simulink subsystem "PvtSubSys_VSM_LKA"  (R2020b)
settings: Solver=VariableStepAuto  StartTime=0.0  StopTime=10.0  RelTol=1e-3
values from neighbouring files (symbols this model uses):
  P_VSM_LKA_AbsEspInTime = 3.0    [LKA.sldd]
  P_VSM_LKA_absLongitudeAcceIn = 2.5    [LKA.sldd]
  P_VSM_LKA_absLongitudeAcceInTime = 3.0    [LKA.sldd]
  P_VSM_LKA_absLongitudeAcceOut = 3.0    [LKA.sldd]
  P_VSM_LKA_AccPedalPosnOut = 30.0    [LKA.sldd]
  P_VSM_LKA_AccPedalRateOutTime = 0.0    [LKA.sldd]
  P_VSM_LKA_AccRateIn = 30.0    [LKA.sldd]
  P_VSM_LKA_AccRateInTime = 1.5    [LKA.sldd]
  P_VSM_LKA_AccRateOut = 70.0    [LKA.sldd]
  P_VSM_LKA_BrakePressIn = 3.0    [LKA.sldd]
  P_VSM_LKA_BrakePressInTime = 1.5    [LKA.sldd]
  P_VSM_LKA_BrakePressOut = 5.0    [LKA.sldd]
  P_VSM_LKA_CurveFactor = 1.0    [LKA.sldd]
  P_VSM_LKA_DriverInputTrqValueIn = 2.0    [LKA.sldd]
  P_VSM_LKA_DriverInputTrqValueInTime = 3.0    [LKA.sldd]
  P_VSM_LKA_DriverInputTrqValueOut = 2.3    [LKA.sldd]
  P_VSM_LKA_EndSwitch = 1.0    [LKA.sldd]
  P_VSM_LKA_LaneChangeOffset = 0.11    [LKA.sldd]
  P_VSM_LKA_LaneCurveIn = 0.005    [LKA.sldd]
  P_VSM_LKA_LaneCurveOut = 0.006    [LKA.sldd]
  P_VSM_LKA_LateralAcceIn = 3.0    [LKA.sldd]
  P_VSM_LKA_LateralAcceInTime = 3.0    [LKA.sldd]
  P_VSM_LKA_LateralAcceOut = 3.5    [LKA.sldd]
  P_VSM_LKA_LongitudeAcceIn = 3.0    [LKA.sldd]
  P_VSM_LKA_LongitudeAcceOut = 3.5    [LKA.sldd]
  P_VSM_LKA_OverrideInTime = 1.5    [LKA.sldd]
  P_VSM_LKA_OverrideTime = 0.3    [LKA.sldd]
  P_VSM_LKA_OverrideValue = 1.2    [LKA.sldd]
  P_VSM_LKA_State_Absesp_enable = 1.0    [LKA.sldd]
  P_VSM_LKA_State_Accpedalrate_enable = 1.0    [LKA.sldd]
  P_VSM_LKA_State_Breakpressure_enable = 1.0    [LKA.sldd]
  P_VSM_LKA_State_DriverInputTrqValue_enable = 1.0    [LKA.sldd]
  P_VSM_LKA_State_Eps_enable = 1.0    [LKA.sldd]
  P_VSM_LKA_State_ESSSts_enable = 1.0    [LKA.sldd]
  P_VSM_LKA_State_Failsafe_enable = 1.0    [LKA.sldd]
  P_VSM_LKA_State_GEAR_enable = 1.0    [LKA.sldd]
  P_VSM_LKA_State_Handson_enable = 1.0    [LKA.sldd]
  P_VSM_LKA_State_Headingangle_enable = 1.0    [LKA.sldd]
  P_VSM_LKA_State_Lane_enable = 1.0    [LKA.sldd]
  P_VSM_LKA_State_LaneChange_enable = 1.0    [LKA.sldd]
  P_VSM_LKA_State_Lanecurve_enable = 1.0    [LKA.sldd]
  P_VSM_LKA_State_LateralAcce_enable = 1.0    [LKA.sldd]
  P_VSM_LKA_State_LongitudeAcc_enable = 1.0    [LKA.sldd]
  P_VSM_LKA_State_Overide_enable = 1.0    [LKA.sldd]
  P_VSM_LKA_State_Param_AngleOffset = 0.15    [LKA.sldd]
  P_VSM_LKA_State_Param_InterventionZoneIn = 0.4    [LKA.sldd]
  P_VSM_LKA_State_Param_InterventionZoneOut = -0.65    [LKA.sldd]
  P_VSM_LKA_State_Param_LaneCurve : value not decoded    [LKA.sldd]
  P_VSM_LKA_State_Param_LaneCurve_Offset : value not decoded    [LKA.sldd]
  P_VSM_LKA_State_Param_LaneWidth_Offset : value not decoded    [LKA.sldd]
  P_VSM_LKA_State_Param_OutOffset = 0.2    [LKA.sldd]
  P_VSM_LKA_State_Param_REInterventionZoneIn = 0.55    [LKA.sldd]
  P_VSM_LKA_State_Param_Sensitive_Offset : value not decoded    [LKA.sldd]
  P_VSM_LKA_State_SteerWheelAngle_enable = 1.0    [LKA.sldd]
  P_VSM_LKA_State_SteerWheelSpd_enable = 1.0    [LKA.sldd]
  P_VSM_LKA_State_TJASts_enable = 1.0    [LKA.sldd]
  P_VSM_LKA_State_TurnLight_enable = 1.0    [LKA.sldd]
  P_VSM_LKA_State_Vehspeed_enable = 1.0    [LKA.sldd]
  P_VSM_LKA_State_Yawsup_enable = 1.0    [LKA.sldd]
  P_VSM_LKA_SteerWheelAngleIn = 70.0    [LKA.sldd]
  P_VSM_LKA_SteerWheelAngleInTime = 3.0    [LKA.sldd]
  P_VSM_LKA_SteerWheelAngleOut = 90.0    [LKA.sldd]
  P_VSM_LKA_SteerWheelSpdIn = 150.0    [LKA.sldd]
  P_VSM_LKA_SteerWheelSpdInTime = 3.0    [LKA.sldd]
  P_VSM_LKA_SteerWheelSpdOut = 200.0    [LKA.sldd]
  P_VSM_LKA_TurnLightInTime = 3.0    [LKA.sldd]
  P_VSM_LKA_Warnarea1 = -0.55    [LKA.sldd]
  P_VSM_LKA_Warnarea2 = -0.35    [LKA.sldd]
  P_VSM_LKA_WarnInTime = 2.0    [LKA.sldd]
  P_VSM_LKA_WhelDy = 2.0    [LKA.sldd]
  P_VSM_LKA_YawRateIn = 0.2    [LKA.sldd]
  P_VSM_LKA_YawRateInTime = 1.0    [LKA.sldd]
  P_VSM_LKA_YawRateOut = 0.25    [LKA.sldd]
undefined symbols (not defined in the file or in its folder): P_VSM_LKA_AddOffset, P_VSM_LSMC_SampleTime, STATE
libraries: simulink x162
(part 4 of 5)

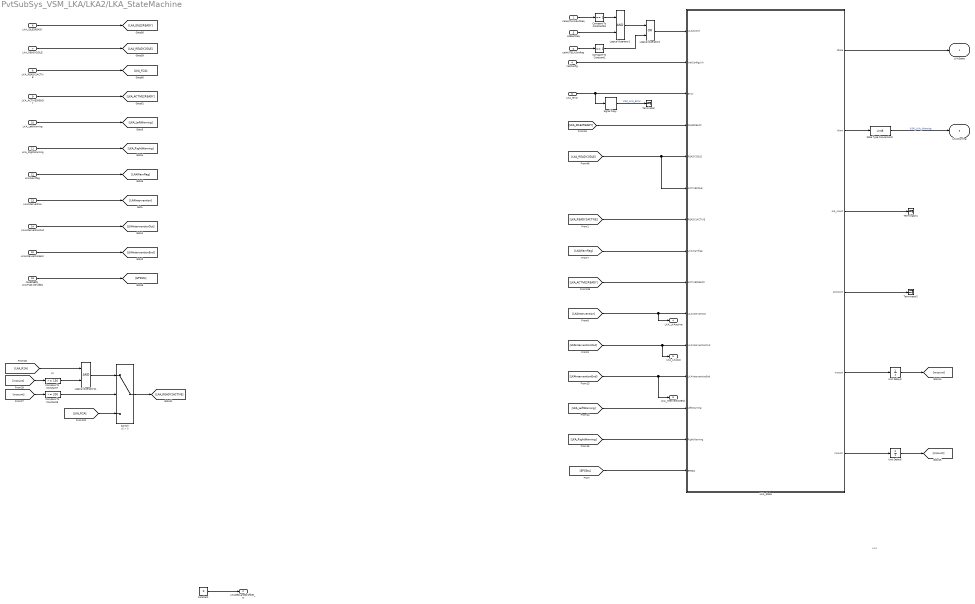
== system PvtSubSys_VSM_LKA/LKA2/LKA_StateMachine ==
  note: 3S
  note: LKA
  canHUTLKASwtReq : Inport
  canHUTELKSwtReq : Inport  Port=2
  LSSSwtReq : Inport  Port=3
  VehConfig : Inport  Port=4
  LKA_Error : Inport  Port=5
  LKA_IDLE2READY : Inport  Port=6
  LKA_READY2IDLE : Inport  Port=7
  LKA_READY2ACTIVE : Inport  Port=8
  LKA_ACTIVE2READY : Inport  Port=9
  LKA_LeftWarning : Inport  Port=10
  LKA_RightWarning : Inport  Port=11
  LKAWarnflag : Inport  Port=12
  LKAIntervention : Inport  Port=13
  LKAInterventionOut : Inport  Port=14
  LKAInterventionEnd : Inport  Port=15
  canEPSEPS_LKATrqOvlDlvdSts : Inport  Port=16
  Compare To Constant1 : simulink/Logic and Bit Operations/Compare To Constant  relop===  const=1  OutDataTypeStr=boolean
  Compare To Constant53 : simulink/Logic and Bit Operations/Compare To Constant  relop===  const=1  OutDataTypeStr=boolean
  Compare To Constant6 : simulink/Logic and Bit Operations/Compare To Constant  relop=>=  const=200  OutDataTypeStr=boolean
  Compare To Constant7 : simulink/Logic and Bit Operations/Compare To Constant  relop=>=  const=150  OutDataTypeStr=boolean
  Constant : Constant  Value=0
  Data Type Conversion2 : DataTypeConversion  OutDataTypeStr=uint8
  LKA_State : Stateflow chart  TreatAsAtomicUnit=on
  Logical Operator1 : Logic  AllPortsSameDT=off  OutDataTypeStr=boolean
  Logical Operator11 : Logic  AllPortsSameDT=off  OutDataTypeStr=boolean
  Logical Operator2 : Logic  Operator=OR  AllPortsSameDT=off  OutDataTypeStr=boolean
  Signal Copy : SignalConversion  OverrideOpt=off
  Switch : Switch  Criteria=u2 > Threshold
  Terminator : Terminator
  Terminator1 : Terminator
  Terminator2 : Terminator
  Unit Delay3 : UnitDelay  SampleTime=-1  HasFrameUpgradeWarning=on
  Unit Delay6 : UnitDelay  SampleTime=-1  HasFrameUpgradeWarning=on
  LKAState : Outport
  LKADesLaneDyoffset_m : Outport  Port=2
  LKAWarning : Outport  Port=3
  LKA_LKAactive : Outport  Port=4
  LKA_LKAout : Outport  Port=5
  LKA_InterventionEnd : Outport  Port=6
  wires:
  Signal Copy/1 -> Terminator/1  "VSM_LKA_Error"
  [EPSSts] -> LKA_State/15(EPSSts)
  canEPSEPS_LKATrqOvlDlvdSts/1 -> [EPSSts]
  LSSSwtReq/1 -> Logical Operator1/2
  Logical Operator2/1 -> LKA_State/1(LKASwitch)
  LKAInterventionEnd/1 -> [LKAInterventionEnd]
  LKAInterventionOut/1 -> [LKAInterventionOut]
  LKAIntervention/1 -> [LKAIntervention]
  LKAWarnflag/1 -> [LKAWarnflag]
  LKA_RightWarning/1 -> [LKA_RightWarning]
  LKA_LeftWarning/1 -> [LKA_LeftWarning]
  Switch/1 -> [LKA_READY2ACTIVE]
  [LKAInterventionEnd] -> LKA_State/12(LKAInterventionEnd), LKA_InterventionEnd/1
  [LKAInterventionOut] -> LKA_State/11(LKAInterventionOut), LKA_LKAout/1
  [LKAIntervention] -> LKA_LKAactive/1, LKA_State/10(LKAIntervention)
  [LKAWarnflag] -> LKA_State/8(LKAWarnflag)
  LKA_State/1(State) -> LKAState/1
  Data Type Conversion2/1 -> LKAWarning/1  "VSM_LKA_Warning"
  LKA_State/4(actcount) -> Terminator2/1
  LKA_State/3(out_count) -> Terminator1/1
  Compare To Constant1/1 -> Logical Operator2/2
  Constant/1 -> LKADesLaneDyoffset_m/1
  [LKA_ACTIVE2READY] -> LKA_State/9(ACTIVE2READY)
  LKA_Error/1 -> LKA_State/3(Error), Signal Copy/1
  [LKA_RightWarning] -> LKA_State/14(RightWarning)
  canHUTLKASwtReq/1 -> Compare To Constant53/1
  [LKA_LeftWarning] -> LKA_State/13(LeftWarning)
  LKA_State/2(Warn) -> Data Type Conversion2/1
  LKA_IDLE2READY/1 -> [LKA_IDLE2READY]
  LKA_READY2IDLE/1 -> [LKA_READY2IDLE]
  LKA_READY2ACTIVE/1 -> [LKA_R2A]
  LKA_ACTIVE2READY/1 -> [LKA_ACTIVE2READY]
  [LKA_IDLE2READY] -> LKA_State/4(IDLE2READY)
  Compare To Constant53/1 -> Logical Operator1/1
  [LKA_READY2IDLE] -> LKA_State/5(READY2IDLE), LKA_State/6(ACTIVE2IDLE)
  LKA_State/5(wcount) -> Unit Delay3/1
  [LKA_R2A] -> Switch/3
  [LKA_READY2ACTIVE] -> LKA_State/7(READY2ACTIVE)
  [LKA_R2A] -> Logical Operator11/1
  Logical Operator11/1 -> Switch/1
  [wcount] -> Compare To Constant6/1
  Compare To Constant6/1 -> Switch/2
  LKA_State/6(incount) -> Unit Delay6/1
  Compare To Constant7/1 -> Logical Operator11/2
  [incount] -> Compare To Constant7/1
  Unit Delay3/1 -> [wcount]
  Unit Delay6/1 -> [incount]
  canHUTELKSwtReq/1 -> Compare To Constant1/1
  Logical Operator1/1 -> Logical Operator2/1
  VehConfig/1 -> LKA_State/2(VehConfigLKA)

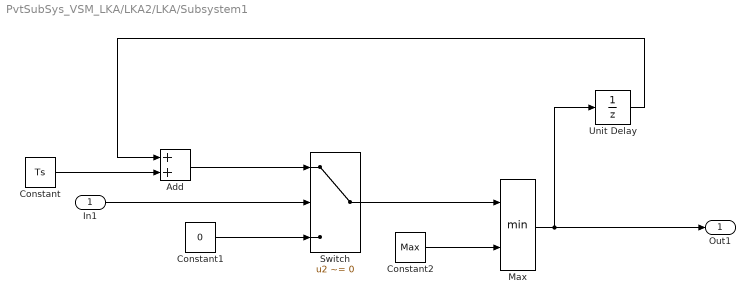
== system PvtSubSys_VSM_LKA/LKA2/LKA/Subsystem1 ==
  In1 : Inport
  Add : Sum
  Constant : Constant  Value=Ts
  Constant1 : Constant  Value=0
  Constant2 : Constant  Value=Max
  Max : MinMax  Inputs=2
  Switch : Switch  Criteria=u2 ~= 0
  Unit Delay : UnitDelay  SampleTime=-1  HasFrameUpgradeWarning=on
  Out1 : Outport
  wires:
  Unit Delay/1 -> Add/1
  In1/1 -> Switch/2
  Constant/1 -> Add/2
  Constant1/1 -> Switch/3
  Add/1 -> Switch/1
  Max/1 -> Unit Delay/1, Out1/1
  Constant2/1 -> Max/2
  Switch/1 -> Max/1

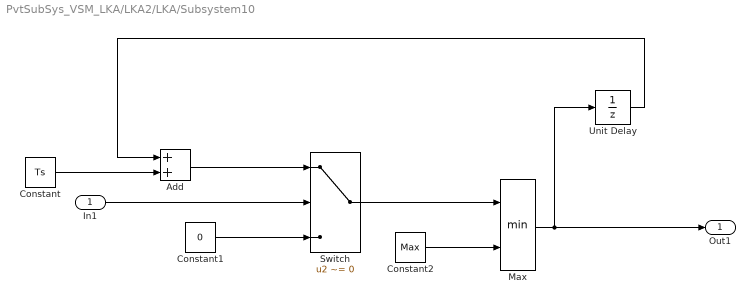
== system PvtSubSys_VSM_LKA/LKA2/LKA/Subsystem10 ==
  In1 : Inport
  Add : Sum
  Constant : Constant  Value=Ts
  Constant1 : Constant  Value=0
  Constant2 : Constant  Value=Max
  Max : MinMax  Inputs=2
  Switch : Switch  Criteria=u2 ~= 0
  Unit Delay : UnitDelay  SampleTime=-1  HasFrameUpgradeWarning=on
  Out1 : Outport
  wires:
  Switch/1 -> Max/1
  Constant2/1 -> Max/2
  Max/1 -> Out1/1, Unit Delay/1
  Add/1 -> Switch/1
  Constant1/1 -> Switch/3
  Constant/1 -> Add/2
  In1/1 -> Switch/2
  Unit Delay/1 -> Add/1

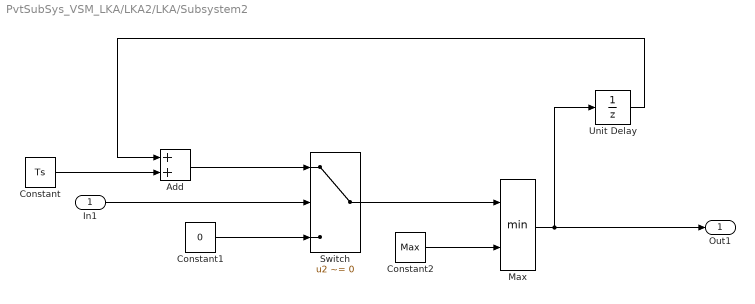
== system PvtSubSys_VSM_LKA/LKA2/LKA/Subsystem2 ==
  In1 : Inport
  Add : Sum
  Constant : Constant  Value=Ts
  Constant1 : Constant  Value=0
  Constant2 : Constant  Value=Max
  Max : MinMax  Inputs=2
  Switch : Switch  Criteria=u2 ~= 0
  Unit Delay : UnitDelay  SampleTime=-1  HasFrameUpgradeWarning=on
  Out1 : Outport
  wires:
  Unit Delay/1 -> Add/1
  In1/1 -> Switch/2
  Constant/1 -> Add/2
  Constant1/1 -> Switch/3
  Add/1 -> Switch/1
  Max/1 -> Unit Delay/1, Out1/1
  Constant2/1 -> Max/2
  Switch/1 -> Max/1

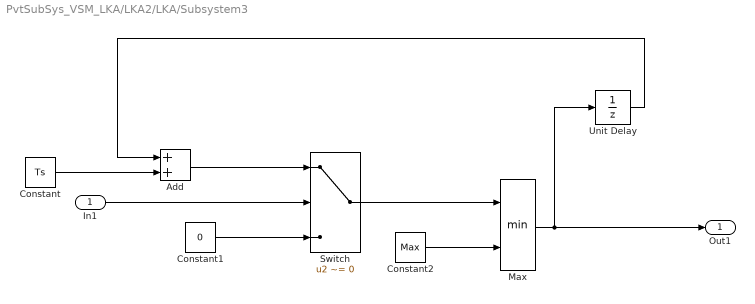
== system PvtSubSys_VSM_LKA/LKA2/LKA/Subsystem3 ==
  In1 : Inport
  Add : Sum
  Constant : Constant  Value=Ts
  Constant1 : Constant  Value=0
  Constant2 : Constant  Value=Max
  Max : MinMax  Inputs=2
  Switch : Switch  Criteria=u2 ~= 0
  Unit Delay : UnitDelay  SampleTime=-1  HasFrameUpgradeWarning=on
  Out1 : Outport
  wires:
  Switch/1 -> Max/1
  Constant2/1 -> Max/2
  Max/1 -> Out1/1, Unit Delay/1
  Add/1 -> Switch/1
  Constant1/1 -> Switch/3
  Constant/1 -> Add/2
  In1/1 -> Switch/2
  Unit Delay/1 -> Add/1

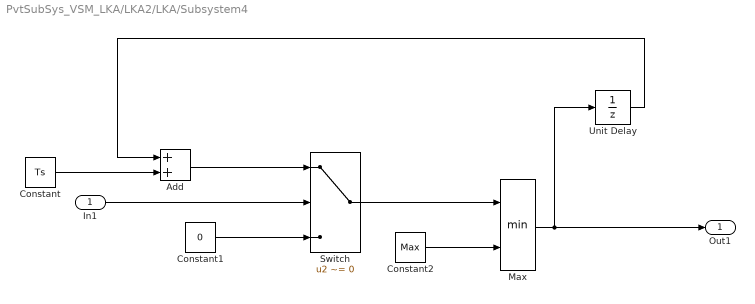
== system PvtSubSys_VSM_LKA/LKA2/LKA/Subsystem4 ==
  In1 : Inport
  Add : Sum
  Constant : Constant  Value=Ts
  Constant1 : Constant  Value=0
  Constant2 : Constant  Value=Max
  Max : MinMax  Inputs=2
  Switch : Switch  Criteria=u2 ~= 0
  Unit Delay : UnitDelay  SampleTime=-1  HasFrameUpgradeWarning=on
  Out1 : Outport
  wires:
  Switch/1 -> Max/1
  Constant2/1 -> Max/2
  Max/1 -> Out1/1, Unit Delay/1
  Add/1 -> Switch/1
  Constant1/1 -> Switch/3
  Constant/1 -> Add/2
  In1/1 -> Switch/2
  Unit Delay/1 -> Add/1

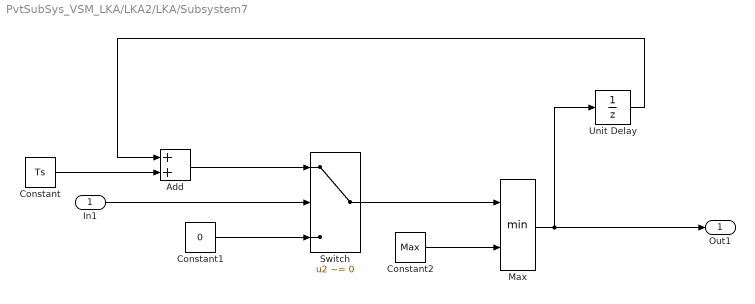
== system PvtSubSys_VSM_LKA/LKA2/LKA/Subsystem7 ==
  In1 : Inport
  Add : Sum
  Constant : Constant  Value=Ts
  Constant1 : Constant  Value=0
  Constant2 : Constant  Value=Max
  Max : MinMax  Inputs=2
  Switch : Switch  Criteria=u2 ~= 0
  Unit Delay : UnitDelay  SampleTime=-1  HasFrameUpgradeWarning=on
  Out1 : Outport
  wires:
  Unit Delay/1 -> Add/1
  In1/1 -> Switch/2
  Constant/1 -> Add/2
  Constant1/1 -> Switch/3
  Add/1 -> Switch/1
  Max/1 -> Unit Delay/1, Out1/1
  Constant2/1 -> Max/2
  Switch/1 -> Max/1

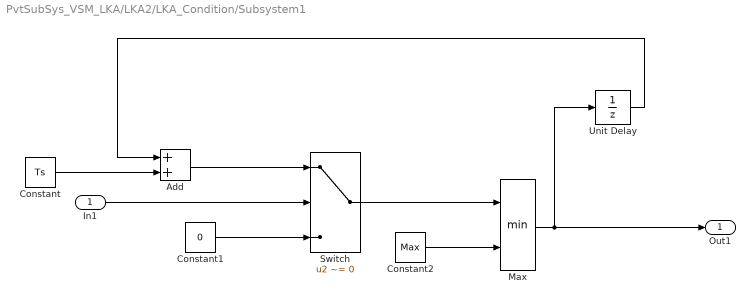
== system PvtSubSys_VSM_LKA/LKA2/LKA_Condition/Subsystem1 ==
  In1 : Inport
  Add : Sum
  Constant : Constant  Value=Ts
  Constant1 : Constant  Value=0
  Constant2 : Constant  Value=Max
  Max : MinMax  Inputs=2
  Switch : Switch  Criteria=u2 ~= 0
  Unit Delay : UnitDelay  SampleTime=-1  HasFrameUpgradeWarning=on
  Out1 : Outport
  wires:
  Unit Delay/1 -> Add/1
  In1/1 -> Switch/2
  Constant/1 -> Add/2
  Constant1/1 -> Switch/3
  Add/1 -> Switch/1
  Max/1 -> Unit Delay/1, Out1/1
  Constant2/1 -> Max/2
  Switch/1 -> Max/1

== system PvtSubSys_VSM_LKA/LKA2/LKA_Condition/Subsystem10 ==
  In1 : Inport
  Add : Sum
  Constant : Constant  Value=Ts
  Constant1 : Constant  Value=0  OutDataTypeStr=single
  Constant2 : Constant  Value=Max  OutDataTypeStr=single
  Max : MinMax  Inputs=2
  Switch : Switch  Criteria=u2 ~= 0
  Unit Delay : UnitDelay  SampleTime=-1  HasFrameUpgradeWarning=on
  Out1 : Outport
  wires:
  Switch/1 -> Max/1
  Constant2/1 -> Max/2
  Max/1 -> Out1/1, Unit Delay/1
  Add/1 -> Switch/1
  Constant1/1 -> Switch/3
  Constant/1 -> Add/2
  In1/1 -> Switch/2
  Unit Delay/1 -> Add/1

== system PvtSubSys_VSM_LKA/LKA2/LKA_Condition/Subsystem12 ==
  In1 : Inport
  Add : Sum
  Constant : Constant  Value=Ts
  Constant1 : Constant  Value=0
  Constant2 : Constant  Value=Max
  Max : MinMax  Inputs=2
  Switch : Switch  Criteria=u2 ~= 0
  Unit Delay : UnitDelay  SampleTime=-1  HasFrameUpgradeWarning=on
  Out1 : Outport
  wires:
  Switch/1 -> Max/1
  Constant2/1 -> Max/2
  Max/1 -> Out1/1, Unit Delay/1
  Add/1 -> Switch/1
  Constant1/1 -> Switch/3
  Constant/1 -> Add/2
  In1/1 -> Switch/2
  Unit Delay/1 -> Add/1

== system PvtSubSys_VSM_LKA/LKA2/LKA_Condition/Subsystem13 ==
  In1 : Inport
  Add : Sum
  Constant : Constant  Value=Ts
  Constant1 : Constant  Value=0
  Constant2 : Constant  Value=Max
  Max : MinMax  Inputs=2
  Switch : Switch  Criteria=u2 ~= 0
  Unit Delay : UnitDelay  SampleTime=-1  HasFrameUpgradeWarning=on
  Out1 : Outport
  wires:
  Switch/1 -> Max/1
  Constant2/1 -> Max/2
  Max/1 -> Out1/1, Unit Delay/1
  Add/1 -> Switch/1
  Constant1/1 -> Switch/3
  Constant/1 -> Add/2
  In1/1 -> Switch/2
  Unit Delay/1 -> Add/1

== system PvtSubSys_VSM_LKA/LKA2/LKA_Condition/Subsystem15 ==
  In1 : Inport
  Add : Sum
  Constant : Constant  Value=Ts
  Constant1 : Constant  Value=0
  Constant2 : Constant  Value=Max
  Max : MinMax  Inputs=2
  Switch : Switch  Criteria=u2 ~= 0
  Unit Delay : UnitDelay  SampleTime=-1  HasFrameUpgradeWarning=on
  Out1 : Outport
  wires:
  Switch/1 -> Max/1
  Constant2/1 -> Max/2
  Max/1 -> Out1/1, Unit Delay/1
  Add/1 -> Switch/1
  Constant1/1 -> Switch/3
  Constant/1 -> Add/2
  In1/1 -> Switch/2
  Unit Delay/1 -> Add/1

== system PvtSubSys_VSM_LKA/LKA2/LKA_Condition/Subsystem18 ==
  In1 : Inport
  Add : Sum
  Constant : Constant  Value=Ts
  Constant1 : Constant  Value=0
  Constant2 : Constant  Value=Max
  Max : MinMax  Inputs=2
  Switch : Switch  Criteria=u2 ~= 0
  Unit Delay : UnitDelay  SampleTime=-1  HasFrameUpgradeWarning=on
  Out1 : Outport
  wires:
  Switch/1 -> Max/1
  Constant2/1 -> Max/2
  Max/1 -> Out1/1, Unit Delay/1
  Add/1 -> Switch/1
  Constant1/1 -> Switch/3
  Constant/1 -> Add/2
  In1/1 -> Switch/2
  Unit Delay/1 -> Add/1

== system PvtSubSys_VSM_LKA/LKA2/LKA_Condition/Subsystem2 ==
  In1 : Inport
  Add : Sum
  Constant : Constant  Value=Ts
  Constant1 : Constant  Value=0
  Constant2 : Constant  Value=Max
  Max : MinMax  Inputs=2
  Switch : Switch  Criteria=u2 ~= 0
  Unit Delay : UnitDelay  SampleTime=-1  HasFrameUpgradeWarning=on
  Out1 : Outport
  wires:
  Switch/1 -> Max/1
  Constant2/1 -> Max/2
  Max/1 -> Out1/1, Unit Delay/1
  Add/1 -> Switch/1
  Constant1/1 -> Switch/3
  Constant/1 -> Add/2
  In1/1 -> Switch/2
  Unit Delay/1 -> Add/1

== system PvtSubSys_VSM_LKA/LKA2/LKA_Condition/Subsystem3 ==
  In1 : Inport
  Add : Sum
  Constant : Constant  Value=Ts
  Constant1 : Constant  Value=0
  Constant2 : Constant  Value=Max
  Max : MinMax  Inputs=2
  Switch : Switch  Criteria=u2 ~= 0
  Unit Delay : UnitDelay  SampleTime=-1  HasFrameUpgradeWarning=on
  Out1 : Outport
  wires:
  Unit Delay/1 -> Add/1
  In1/1 -> Switch/2
  Constant/1 -> Add/2
  Constant1/1 -> Switch/3
  Add/1 -> Switch/1
  Max/1 -> Unit Delay/1, Out1/1
  Constant2/1 -> Max/2
  Switch/1 -> Max/1

== system PvtSubSys_VSM_LKA/LKA2/LKA_Condition/Subsystem4 ==
  In1 : Inport
  Add : Sum
  Constant : Constant  Value=Ts
  Constant1 : Constant  Value=0
  Constant2 : Constant  Value=Max
  Max : MinMax  Inputs=2
  Switch : Switch  Criteria=u2 ~= 0
  Unit Delay : UnitDelay  SampleTime=-1  HasFrameUpgradeWarning=on
  Out1 : Outport
  wires:
  Switch/1 -> Max/1
  Constant2/1 -> Max/2
  Max/1 -> Out1/1, Unit Delay/1
  Add/1 -> Switch/1
  Constant1/1 -> Switch/3
  Constant/1 -> Add/2
  In1/1 -> Switch/2
  Unit Delay/1 -> Add/1

== system PvtSubSys_VSM_LKA/LKA2/LKA_Condition/Subsystem5 ==
  In1 : Inport
  Add : Sum
  Constant : Constant  Value=Ts
  Constant1 : Constant  Value=0
  Constant2 : Constant  Value=Max
  Max : MinMax  Inputs=2
  Switch : Switch  Criteria=u2 ~= 0
  Unit Delay : UnitDelay  SampleTime=-1  HasFrameUpgradeWarning=on
  Out1 : Outport
  wires:
  Unit Delay/1 -> Add/1
  In1/1 -> Switch/2
  Constant/1 -> Add/2
  Constant1/1 -> Switch/3
  Add/1 -> Switch/1
  Max/1 -> Unit Delay/1, Out1/1
  Constant2/1 -> Max/2
  Switch/1 -> Max/1

== system PvtSubSys_VSM_LKA/LKA2/LKA_Condition/Subsystem6 ==
  In1 : Inport
  Add : Sum
  Constant : Constant  Value=Ts
  Constant1 : Constant  Value=0
  Constant2 : Constant  Value=Max
  Max : MinMax  Inputs=2
  Switch : Switch  Criteria=u2 ~= 0
  Unit Delay : UnitDelay  SampleTime=-1  HasFrameUpgradeWarning=on
  Out1 : Outport
  wires:
  Unit Delay/1 -> Add/1
  In1/1 -> Switch/2
  Constant/1 -> Add/2
  Constant1/1 -> Switch/3
  Add/1 -> Switch/1
  Max/1 -> Unit Delay/1, Out1/1
  Constant2/1 -> Max/2
  Switch/1 -> Max/1

== system PvtSubSys_VSM_LKA/LKA2/LKA_Condition/Subsystem7 ==
  In1 : Inport
  Add : Sum
  Constant : Constant  Value=Ts
  Constant1 : Constant  Value=0
  Constant2 : Constant  Value=Max
  Max : MinMax  Inputs=2
  Switch : Switch  Criteria=u2 ~= 0
  Unit Delay : UnitDelay  SampleTime=-1  HasFrameUpgradeWarning=on
  Out1 : Outport
  wires:
  Switch/1 -> Max/1
  Constant2/1 -> Max/2
  Max/1 -> Out1/1, Unit Delay/1
  Add/1 -> Switch/1
  Constant1/1 -> Switch/3
  Constant/1 -> Add/2
  In1/1 -> Switch/2
  Unit Delay/1 -> Add/1

== system PvtSubSys_VSM_LKA/LKA2/LKA_Condition/Subsystem8 ==
  In1 : Inport
  Add : Sum
  Constant : Constant  Value=Ts
  Constant1 : Constant  Value=0
  Constant2 : Constant  Value=Max
  Max : MinMax  Inputs=2
  Switch : Switch  Criteria=u2 ~= 0
  Unit Delay : UnitDelay  SampleTime=-1  HasFrameUpgradeWarning=on
  Out1 : Outport
  wires:
  Unit Delay/1 -> Add/1
  In1/1 -> Switch/2
  Constant/1 -> Add/2
  Constant1/1 -> Switch/3
  Add/1 -> Switch/1
  Max/1 -> Unit Delay/1, Out1/1
  Constant2/1 -> Max/2
  Switch/1 -> Max/1

== system PvtSubSys_VSM_LKA/LKA2/LKA_Condition/Subsystem9 ==
  In1 : Inport
  Add : Sum
  Constant : Constant  Value=Ts
  Constant1 : Constant  Value=0
  Constant2 : Constant  Value=Max
  Max : MinMax  Inputs=2
  Switch : Switch  Criteria=u2 ~= 0
  Unit Delay : UnitDelay  SampleTime=-1  HasFrameUpgradeWarning=on
  Out1 : Outport
  wires:
  Switch/1 -> Max/1
  Constant2/1 -> Max/2
  Max/1 -> Out1/1, Unit Delay/1
  Add/1 -> Switch/1
  Constant1/1 -> Switch/3
  Constant/1 -> Add/2
  In1/1 -> Switch/2
  Unit Delay/1 -> Add/1

== matlab function PvtSubSys_VSM_LKA/LKA2/LKA_Condition/MATLAB Function ==
  data: LeftChangefg input; y output; RightChangefg input; Ldy input; Rdy input; Lfgk1 input; Lfg output; Rfgk1 input; Rfg output
function [y,Lfg,Rfg] = fcn(LeftChangefg,RightChangefg,Ldy,Rdy,Lfgk1,Rfgk1)
y=1;
Lfg=0;
Rfg=0;
if LeftChangefg>0
    Lfg=1;
    y=0;
elseif Lfgk1>0
    Lfg=1;
    y=0;
    if Rdy>0
        Lfg=0;
        y=1;
    end
    
end

if RightChangefg>0
    Rfg=1;
    y=0;
elseif Rfgk1>0
    Rfg=1;
    y=0;
    if Ldy>0
        Rfg=0;
        y=1;
    end
    
end

== matlab function PvtSubSys_VSM_LKA/LKA2/LKA_Condition/State_TurnLight2 ==
  data: leftlight input; rightlight input; lane input; state output; out output; leftk1 input; left output; rightk1 input; right output
function [state,out,left,right] = fcn(leftlight,rightlight,lane,leftk1,rightk1)
left=0;
right=0;
if leftlight==1 && lane==1  % left alone
    state=1;
    out=0;
    left=1;
elseif lane==1 && leftk1==1  
    state=0;
    out=0;
    left=1;
elseif lane ==1
    state=0;
    out=1;
    left=0;
elseif rightlight==1 && lane==2
    state=1;
    out=0;
    right=1;
elseif lane==2 && rightk1==1
    state=0;
    out=0;
    right=1;
elseif lane ==2
    state=0;
    out=1;
    right=0;
    
else
    state=0;
    out=0;
    left=0;
end

== stateflow chart PvtSubSys_VSM_LKA/LKA2/LKA_StateMachine/LKA_State ==
  state MAINST_ERROR
    en:State=STATE.ERROR
  state MAINST_OFF
    en:State=STATE.OFF;
  state MAINST_ON
    state SUBST_IDLE
      en:State=STATE.IDLE;
    state SUBST_ACTIVE
      state SUBST_ACTIVE_LEFT
        en:State=STATE.ACTIVE_LEFT;
        actcount=0;
        incount=0;
        du:
        actcount = actcount + 1;
        state LEFT_ACTIVE
          en:wcount=0;
          du:
          if LKAInterventionOut==1
          out_count=out_count+1;
          else
          out_count=0;
          end
        state LEFT_WARN
          en:Warn=1;wcount=0;
          du:wcount=wcount+1;
          ex:Warn=0;
        LEFT_ACTIVE -> LEFT_WARN : [LeftWarning==true || (actcount>50*20 && out_count<10)]
        LEFT_WARN -> LEFT_ACTIVE : [ LeftWarning==false && actcount<50*20 ]
      state SUBST_ACTIVE_RIGHT
        en:State=STATE.ACTIVE_RIGHT;
        actcount=0;
        incount=0;
        du:
        actcount = actcount + 1;
        state RIGHT_ACTIVE
          en:wcount=0;
          du:
          if LKAInterventionOut==1
          out_count=out_count+1;
          else
          out_count=0;
          end
        state RIGHT_WARN
          en:Warn=1;wcount=0;
          du:wcount=wcount+1;
          ex:Warn=0;
        RIGHT_ACTIVE -> RIGHT_WARN : [RightWarning==true || (actcount>50*20 && out_count<10)]
        RIGHT_WARN -> RIGHT_ACTIVE : [RightWarning==false && actcount<50*20]
      (junction 37) -> LEFT_ACTIVE [order 1] : [LKAIntervention==1]
      (junction 37) -> RIGHT_ACTIVE [order 2] : [LKAIntervention==2]
    state SUBST_READY
      en:State=STATE.READY;actcount=0;
      out_count=0;
      du:
      if wcount>=4*50
      incount=incount+1;
      else
      incount=0;
      end
    (default) -> SUBST_IDLE
    SUBST_IDLE -> SUBST_READY : [IDLE2READY && LKAWarnflag==1 && Error~=3]
    SUBST_READY -> SUBST_IDLE [order 2] : [READY2IDLE || Error==3]
    SUBST_ACTIVE -> SUBST_IDLE : [ACTIVE2IDLE || Error==3]
    SUBST_ACTIVE_LEFT -> SUBST_READY : [ACTIVE2READY ||...
        | LKAInterventionEnd==1||...
        | wcount>=4*50||out_count>=1.5*50]
    SUBST_READY -> (junction 37) [order 1] : [READY2ACTIVE]
    SUBST_ACTIVE_RIGHT -> SUBST_READY : [ACTIVE2READY||...
        | LKAInterventionEnd==1||...
        | wcount>=4*50||out_count>=1.5*50]
  (default) -> MAINST_OFF
  MAINST_OFF -> MAINST_ERROR [order 1] : [LKASwitch==true&&Error==1&& VehConfigLKA==1]
  MAINST_ERROR -> MAINST_OFF [order 1] : [LKASwitch==false]
  MAINST_OFF -> MAINST_ON [order 2] : [LKASwitch==true && VehConfigLKA==1]
  MAINST_ON -> MAINST_OFF [order 1] : [LKASwitch==false]
  MAINST_ERROR -> MAINST_ON [order 2] : [LKASwitch==true && Error~=1 && EPSSts~=3]
  MAINST_ON -> MAINST_ERROR [order 2] : [Error==1 || EPSSts==3]
  data: LKASwitch input; VehConfigLKA input uint8; Error input; IDLE2READY input; READY2IDLE input; ACTIVE2IDLE input; READY2ACTIVE input; LKAWarnflag input; ACTIVE2READY input; State output Enum: STATE =STATE.OFF; LKAIntervention input; LKAInterventionOut input; LKAInterventionEnd input; LeftWarning input; RightWarning input; Warn output =0; out_count output =0; actcount output; wcount output =0; incount output =0; EPSSts input

== matlab function PvtSubSys_VSM_LKA/LKA2/LKA_Condition/MATLAB Function1 ==
  data: HandsOff_Ready2Idle input; y output; LKASts input; yK1 input
function y = fcn(HandsOff_Ready2Idle, LKASts,yK1)
y=0;
if LKASts==1
    if HandsOff_Ready2Idle==1
        y=1;
    else
        y=yK1;
    end
elseif LKASts~=1
    y=0;
end

== matlab function PvtSubSys_VSM_LKA/LKA2/LKA/MATLAB Function2 ==
  data: T_A2 input; Offset output; LaneCurveOffset input
function Offset = fcn(T_A2, LaneCurveOffset)
Offset=0;
if T_A2>0
    Offset=LaneCurveOffset;
elseif T_A2<0
    Offset=-LaneCurveOffset;
end

== matlab function PvtSubSys_VSM_LKA/LKA2/LKA/MATLAB Function3 ==
  data: active_fg input; PreFLWhelDy input; PreFRWhelDy input; FLWhelDy input; FRWhelDy input; Left_Valid input; Right_Valid input; OutOffset input; LKA_active output single; LKA_Out output single; LKA_End output single; leftactive output; rightactive output; ReactionZoneInDy_m input; ReactionZoneOutDy_m input; Angleoffset input; TargetLine input; HeadingAngel input; LaneCurveOffset input; lfgk1 input; lfg output single; loutk1 input; lout output single; rfgk1 input; routk1 input; rfg output single; rout output single
function [LKA_active,LKA_Out,LKA_End,leftactive,rightactive, lfg,lout,rfg,rout]  = fcn(active_fg,PreFLWhelDy,PreFRWhelDy,FLWhelDy,FRWhelDy,......
    Left_Valid,Right_Valid,OutOffset,ReactionZoneInDy_m,ReactionZoneOutDy_m,Angleoffset,TargetLine,HeadingAngel,LaneCurveOffset, lfgk1,loutk1,rfgk1,routk1)

LKA_active=single(0);
LKA_Out=single(0);
LKA_End=single(0);
lfg=single(0);
rfg=single(0);
lout=single(0);
rout=single(0);
leftactive=ReactionZoneInDy_m-LaneCurveOffset;
rightactive=ReactionZoneInDy_m+LaneCurveOffset;
if Left_Valid>0 && active_fg==single(1) 
    if  PreFLWhelDy<(ReactionZoneInDy_m-LaneCurveOffset) && PreFLWhelDy>(ReactionZoneOutDy_m-LaneCurveOffset) % 进入区域 -0.9--0.4
        if loutk1==single(1)
            lout=single(1);
            LKA_End=single(0);
            lfg=single(0);
        else
            LKA_active= single(1);
            lfg=single(1);
            lout=single(0);
        end
    elseif TargetLine<-OutOffset  &&  FLWhelDy>ReactionZoneOutDy_m && lfgk1>0 %扩大
        if loutk1==single(1)
            lout=single(1);
            LKA_End=single(0);
            lfg=single(0);
        else
            LKA_active= single(1);
            lfg=single(1);
            lout=single(0);
        end
    elseif TargetLine>-OutOffset && TargetLine<OutOffset && HeadingAngel>-Angleoffset && HeadingAngel< Angleoffset%稳定保持退出
        if loutk1==single(1)
            lout=single(1);
            LKA_End=single(0);
            lfg=single(0);
        else
            lfg=single(0);
            lout=single(0);
            LKA_Out=single(1);
        end

         
    elseif FLWhelDy < ReactionZoneOutDy_m   % 驶出 -0.9m
        lout=single(1);
        LKA_End=single(1);
    elseif FLWhelDy > ReactionZoneInDy_m + 0.1  
        lout=single(0);
   
         
    end
end

if Right_Valid>single(0) && active_fg==single(1)
    if  PreFRWhelDy<(ReactionZoneInDy_m+LaneCurveOffset) && PreFRWhelDy>(ReactionZoneOutDy_m+LaneCurveOffset) % 进入区域
        if routk1==single(1)
            rout=single(1);
            LKA_End=single(0);
            rfg=single(0);
        else
            LKA_active= single(2);
            rfg=single(1);
            rout=single(0);
        end
    elseif TargetLine<-OutOffset  &&  FRWhelDy>ReactionZoneOutDy_m && rfgk1>0
        if routk1==single(1)
            rout=single(1);
            LKA_End=single(0);
            rfg=single(0);
        else
            LKA_active= single(2);
            rfg=single(1);
            rout=single(0);
        end
    elseif TargetLine>-OutOffset && TargetLine<OutOffset && HeadingAngel>-Angleoffset && HeadingAngel< Angleoffset
        if routk1==single(1)
            rout=single(1);
            LKA_End=single(0);
            rfg=single(0);
        else
            rfg=single(0);
            rout=single(0);
            LKA_Out=single(1);
        end

         
    elseif FRWhelDy < ReactionZoneOutDy_m   % 驶出 -0.9m
        rout=single(1);
        LKA_End=single(1);
    elseif FRWhelDy > ReactionZoneInDy_m+0.1
        rout=single(0);
    
        
    end
end

if Left_Valid==single(0) && Right_Valid==single(0)
    LKA_End=single(1);
end

== matlab function PvtSubSys_VSM_LKA/LKA2/LKA/MATLAB Function ==
  data: ReactionZoneInDy_m input double size=1; Warnflag output single size=1; preFLWhelDy input single size=1; preFRWhelDy input single size=1
function Warnflag = fcn(ReactionZoneInDy_m, preFLWhelDy, preFRWhelDy)

 if  preFLWhelDy<ReactionZoneInDy_m && preFLWhelDy>-20   % 进入区域
     Warnflag=single(0);
 elseif preFRWhelDy<ReactionZoneInDy_m && preFRWhelDy>-20 % 进入区域
     Warnflag=single(0);
 else
     Warnflag=single(1);
 end
